simulink library "THB_WetBulbTemperature"  (R2018b)
settings: Solver=ode45  StartTime=0.0  StopTime=10.0  RelTol=1e-3  EnableMultiTasking=on
libraries: carnot x2, simulink x1
settings Model: Creator=lena.frank  LastModifiedBy=drhf
settings DataIOCC: LimitDataPoints=on  SaveFormat=Array  SignalLoggingSaveFormat=ModelDataLogs
settings OptimizationCC: ExpressionDepthLimit=2147483647  LifeSpan=inf
settings DebuggingCC: UnderspecifiedInitializationDetection=Classic  MergeDetectMultiDrivingBlocksExec=none  SolverPrmCheckMsg=warning  FcnCallInpInsideContextMsg=warning  StateNameClashWarn=warning  SFUnexpectedBacktrackingDiag=warning  SFNoUnconditionalDefaultTransitionDiag=warning  SFExecutionAtInitializationDiag=none
settings HardwareCC: ProdBitPerPointer=32  ProdBitPerSizeT=32  ProdBitPerPtrDiffT=32  ProdLargestAtomicFloat=None  ProdIntDivRoundTo=Undefined  ProdEndianess=Unspecified  ProdWordSize=32  ProdHWDeviceType=32-bit Generic
settings ModelReferenceCC: PropagateSignalLabelsOutOfModel=off
settings SFSimCC: SimUseLocalCustomCode=off
settings RTWCC: RTWUseLocalCustomCode=off
settings CodeAppCC: StateflowObjectComments=on
settings GRTTargetCC: TargetLangStandard=C89/C90 (ANSI)  GeneratePreprocessorConditionals=Disable all  CombineOutputUpdateFcns=off  GRTInterface=on
settings ConfigComp: CovMetricSettings=dw  CovHtmlReporting=on  CovSaveCumulativeToWorkspaceVar=on  CovSaveSingleToWorkspaceVar=on  CovExternalEMLEnable=off

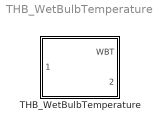
== system THB_WetBulbTemperature ==
  THB_WetBulbTemperature : Subsystem  mask(THB to wet bulb temperature and relative humidity){}
      mask help:
      | Calculate  - the relative humidity of air (rH)
      |                  - and the wet bulb temperature of air (WBT)
      | from          - dry bulb air temperature (DBT)
      |                  - and mass of water per mass of air (x)
      | in THV vector.
      |
      | DBT        [degree centigrade]
      | p              [Pa]
      | x              kg water / kg air
      |
      | rel_hum   [percent]
      | WBT       [degree centigrade] -> T_WBT is valid for T [-6..40°C]
      mask Help: web(fullfile(path_carnot('help'),'THB_Wet_BulbTemperature.html'),'-helpbrowser')

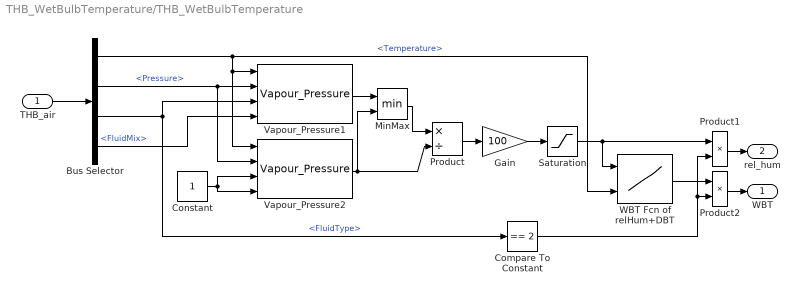
== system THB_WetBulbTemperature/THB_WetBulbTemperature ==
  THB_air : Inport
  Bus Selector : BusSelector  OutputSignals=Temperature,Pressure,FluidType,FluidMix
  Compare To Constant : simulink/Logic and Bit Operations/Compare To Constant  relop===  const=2  OutDataTypeStr=uint8  ZeroCross=off
  Constant : Constant
  Gain : Gain  Gain=100
  MinMax : MinMax  Inputs=2
  Product : Product  Inputs=*/  RndMeth=Zero
  Product1 : Product  RndMeth=Zero
  Product2 : Product  RndMeth=Zero
  Saturation : Saturate  UpperLimit=100  LowerLimit=0
  Vapour_Pressure1 : carnot/Basic/Material_Properties/Vapour_Pressure  VariantControl=CarlibClassic  INPUTARGUMENTS=state variables (classic)  DEBUGLEVEL=WARNINGLEVEL  MAXTOTALMESSAGES=inf  MAXCONSECUTIVEMESSAGES=inf  WRITETOFILE=0  FILENAME='errors.txt'
      settings: SourceProductName=Carnot
  Vapour_Pressure2 : carnot/Basic/Material_Properties/Vapour_Pressure  VariantControl=CarlibClassic  INPUTARGUMENTS=state variables (classic)  DEBUGLEVEL=WARNINGLEVEL  MAXTOTALMESSAGES=inf  MAXCONSECUTIVEMESSAGES=inf  WRITETOFILE=0  FILENAME='errors.txt'
      settings: SourceProductName=Carnot
  WBT Fcn of relHum+DBT : Lookup2D  RowIndex=[0,5,10,15,20,25,30,35,40,45,50,55,60,65,70,75,80,85,90,95,100]  ColumnIndex=[-6,-4,-2,0,2,4,6,8,10,12,14,16,18,20,22,24,26,28,30,32,34,36,38,40]  Table=reshape([-10.3,-10.1,-9.9,-9.3,-9.3,-8.9,-8.8,-8.8,-8.3,-8.2,-8.2,-7.7,-7.7,-7.7,-7.1,-7.1,-7.1,-6.6,-6.6,-6.0,-6,-8.3,-8.1,-7.9,-7.9,-7.8,-7.3,-7.3,-6.8,-6.8,-6.7,-6.2,-6.2,-5.7,-5.7,-5.6,-5.1,-5.1,-4.6,-4.6,-4.6,-4,-7.2,-6.9,-6.7,-6.4,-6.1,-5.9,-5.6,-5.3,-5.0,-4.8,-4.8,-4.2,-4.2,-3.7,-3.7,-3.1,-3.1,-2.6,-2.6,-2.6,-2,-5.6,-5.3,-5.0,-5.0,-4.4,-4.4,-3.9,-3.9,-3.3,-3.3,-2.8,-2.8,-2.2,-2.2,-1.7,-1.7,-1.1,-1.1,-0.6,-0.6,0,-4.5,-4.2,-3.9,-3.6,-3.0,-2.8,-2.4,-1.9,-1.9,-1.3,-1.3,-0.8,-0.6,-0.2,0.1,0.4,0.7,1.1,1.4,1.7,2,-3.4,-3.0,-2.7,-2.1,-1.6,-1.1,-1.0,-0.4,0.0,0.1,0.5,0.8,1.2,1.6,1.9,2.3,2.6,3.0,3.3,3.7,4,-1.9,-1.5,-1.1,-0.7,-0.3,0.1,0.5,0.9,1.3,1.8,2.2,2.6,3.0,3.4,3.8,4.1,4.5,4.9,5.3,5.6,6,-0.8,-0.4,0.1,0.6,1.1,1.5,2.0,2.5,2.9,3.4,3.8,4.3,4.7,5.1,5.6,6.0,6.4,6.8,7.2,7.6,8,0.3,0.8,1.4,1.9,2.5,3.0,3.5,4.0,4.5,5.0,5.5,6.0,6.5,6.9,7.4,7.8,8.3,8.7,9.2,9.6,10,1.4,2.1,2.7,3.3,3.9,4.4,5.0,5.6,6.1,6.6,7.2,7.7,8.2,8.7,9.2,9.7,10.2,10.6,11.1,11.6,12,2.6,3.2,3.9,4.6,5.2,5.8,6.5,7.1,7.7,8.2,8.8,9.4,9.9,10.5,11.0,11.5,12.0,12.5,13.0,13.5,14,3.7,4.4,5.1,5.9,6.6,7.3,7.9,8.6,9.2,9.9,10.5,11.1,11.7,12.2,12.8,13.4,13.9,14.5,15.0,15.5,16,4.7,5.5,6.3,7.1,7.9,8.6,9.4,10.1,10.8,11.5,12.1,12.8,13.4,14.0,14.6,15.2,15.8,16.4,16.9,17.5,18,5.7,6.6,7.5,8.4,9.2,10.0,10.8,11.6,12.3,13.1,13.8,14.5,15.1,15.8,16.4,17.1,17.7,18.3,18.9,19.4,20,6.7,7.7,8.7,9.6,10.5,11.4,12.2,13.1,13.9,14.6,15.4,16.1,16.9,17.6,18.2,18.9,19.6,20.2,20.8,21.4,22,7.7,8.8,9.8,10.8,11.8,12.8,13.7,14.6,15.4,16.2,17.0,17.8,18.6,19.3,20.1,20.8,21.4,22.1,22.7,23.4,24,8.6,9.8,11.0,12.1,13.1,14.1,15.1,16.0,17.0,17.8,18.7,19.5,20.3,21.1,21.9,22.6,23.3,24.0,24.7,25.4,26,9.6,10.8,12.1,13.3,14.4,15.5,16.5,17.5,18.5,19.4,20.3,21.2,22.1,22.9,23.7,24.5,25.2,25.9,26.6,27.3,28,10.4,11.8,13.2,14.4,15.7,16.8,17.9,19.0,20.0,21.0,22.0,22.9,23.8,24.7,25.5,26.3,27.1,27.8,28.6,29.3,30,11.3,12.8,14.3,15.6,16.9,18.2,19.4,20.5,21.6,22.6,23.6,24.6,25.5,26.4,27.3,28.2,29.0,29.8,30.5,31.3,32,12.1,13.8,15.3,16.8,18.2,19.5,20.8,22.0,23.1,24.2,25.3,26.3,27.3,28.2,29.1,30.0,30.9,31.7,32.5,33.3,34,12.9,14.7,16.4,18.0,19.5,20.9,22.2,23.5,24.7,25.9,27.0,28.0,29.0,30.0,31.0,31.9,32.8,33.6,34.4,35.2,36,13.7,15.7,17.5,19.1,20.7,22.2,23.6,25.0,26.3,27.5,28.6,29.7,30.8,31.8,32.8,33.7,34.7,35.5,36.4,37.2,38,14.5,16.6,18.5,20.3,22.0,23.6,25.1,26.5,27.8,29.1,30.3,31.5,32.6,33.6,34.6,35.6,36.6,37.5,38.3,39.2,40],21,24)  RndMeth=Nearest  LUTDesignDataSource=Matlab Workspace  LUTDesignUseExistingBP=off  LUTDesignAbsError=NaN
  WBT : Outport
  rel_hum : Outport  Port=2
  wires:
  THB_air/1 -> Bus Selector/1
  Bus Selector/2 -> Vapour_Pressure2/2, Vapour_Pressure1/2  "<Pressure>"
  Bus Selector/3 -> Vapour_Pressure1/3, Compare To Constant/1  "<FluidType>"
  Bus Selector/4 -> Vapour_Pressure1/4  "<FluidMix>"
  Bus Selector/1 -> WBT Fcn of relHum+DBT/2, Vapour_Pressure2/1, Vapour_Pressure1/1  "<Temperature>"
  Constant/1 -> Vapour_Pressure2/4, Vapour_Pressure2/3
  Vapour_Pressure1/1 -> MinMax/1
  Vapour_Pressure2/1 -> MinMax/2, Product/2
  MinMax/1 -> Product/1
  Product/1 -> Gain/1
  WBT Fcn of relHum+DBT/1 -> Product2/1
  Gain/1 -> Saturation/1
  Saturation/1 -> WBT Fcn of relHum+DBT/1, Product1/1
  Product1/1 -> rel_hum/1
  Product2/1 -> WBT/1
  Compare To Constant/1 -> Product2/2, Product1/2
